simulink model "acc_test"  (R2020a)
settings: Solver=VariableStepAuto  StartTime=0.0  StopTime=6594  RelTol=1e-3
values from neighbouring files (symbols this model uses):
  max_CE_power = 100    [Parallel_script.m]    (also in Series_script.m = 60)
  max_EG_power = 40    [Series_script.m]
  max_EM_power = 84    [Parallel_script.m]    (also in Series_script.m = 90)
  max_SOC = 0.60    (= 0.6)    [Parallel_script.m]    (also in Series_script.m = 0.5)
  min_SOC = 0.35    [Parallel_script.m]    (also in Series_script.m = 0.3)
  Series_add_Mass = 150    [Series_script.m]
  T_CE_max = p_me_max*V_d/(2*pi*2)    [Parallel_script.m]    (also in Series_script.m)
  T_EG_max = T_EG_max * max_EG_power*1000/max_EG_power_old    [Series_script.m]
  T_EM_max = T_EM_max * max_EM_power*1000/max_EM_power_old    [Parallel_script.m]    (also in Series_script.m)
  V_Mass = 1920    [Parallel_script.m]    (also in Series_script.m)
undefined symbols (not defined in the file or in its folder): eta_EG_map, eta_EM_map, H_u, P_aux, P_CE_cutoff, P_CE_idle, T_CE_cutoff, theta_CE, theta_EM, V_CE_map, w_CE_idle, w_CE_max, w_CE_upper, w_EG_row, w_EG_upper, w_EM_row, w_EM_upper
libraries: qss_tb_library x7
settings Model: Creator=Rahul Pai  LastModifiedBy=Rahul Pai

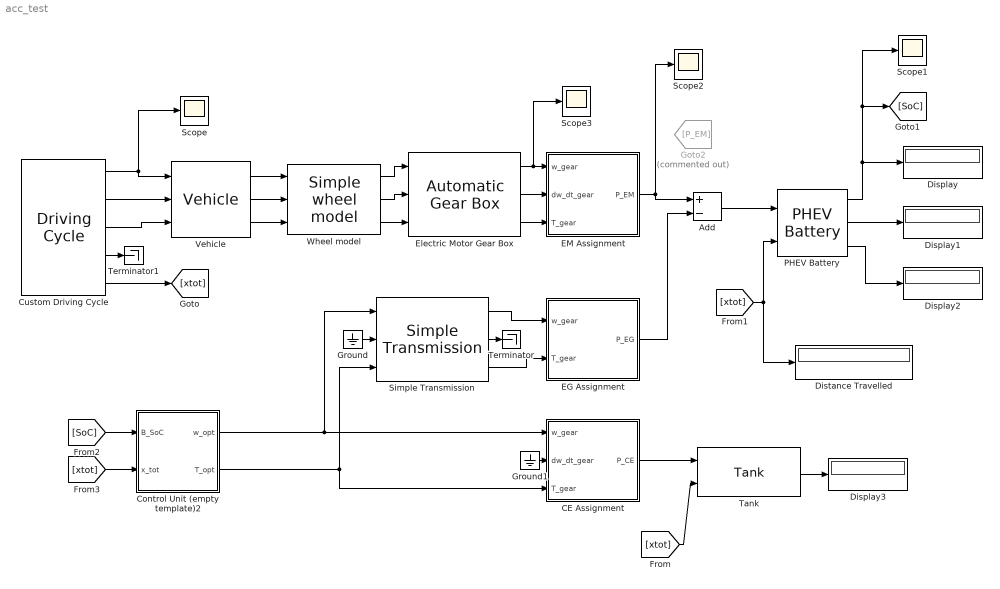
== system acc_test ==
  Add : Sum  Inputs=+-
  CE Assignment : Subsystem  Tag=combustion engine  AncestorBlock=qss_tb_library/Energy Converter/CE Assignment  mask(Combustion Engine (based on consumption map)){engine_type=Gasoline, P_ice=max_CE_power, ENABLE_FUEL_CUTOFF=on}
      mask prompts: engine_type "Engine type"; P_ice "Power [kW]"; ENABLE_FUEL_CUTOFF "Enable fuel cutoff"
      mask help:
      | This block simulates the behaviour of a combustion engine. The block is based on consumption maps for medium sized passenger cars.
      |
      | NA Gasoline:
      | max power @ 5000 rpm
      | max torque @ 3000 rpm
      |
      | Small Diesel:
      | max power @ 4500 rpm
      | max torque @ 2000 rpm
      |
      | Large Diesel:
      | max power @ 1500 rpm
      | max torque @ 1500 rpm
      |
      |
      | Input:
      | =====
      | 	w_gear	Speed of the fly wheel [rad/s]
      | 	dw_dt_gear	Acceleration of the fly wheel [rad/s^2]
      | 	T_gear	Torque on the fly wheel [Nm]
      |
      | Output:
      | ======
      | 	P_CE	Fuel power consumed by the combustion engine [W]
      mask init:
      | init_AssCE_map;
      mask TypeOptions engine_type: Gasoline | Small Diesel | Large Diesel
  Control Unit (empty template)2 : Subsystem  Tag=control unit  AncestorBlock=|  mask(Control Unit){}
      | qss_tb_library/Controller/Control Unit
      | (empty template)
      mask help:
      | This block gives the user the opportunity to design his/her own control unit.
      |
      | The user can define the inputs and outputs  by himself/herself.
  Custom Driving Cycle : qss_tb_library/Driving Cycle/Driving Cycle  Tag=cycle  cyclename1=assignment2_custom_cycle_full  stepsize=1  autostop=on
  Display{,1..3} (4 alike) : Display
  Distance Travelled : Display
      settings: Format=decimal (Stored Integer)
  EG Assignment : Subsystem  AncestorBlock=qss_tb_library/Energy Converter/EG Assignment  mask(Electric Generator){P_eg=max_EG_power}
      mask prompts: P_eg "Maximum mechanical power [kW]"
      mask help:
      | This block simulates the behaviour of an electric generator. The block is based on an efficiency map.
      |
      | Input:
      | =====
      | 	w_gear	Speed of the generator [rad/s]
      | 	T_gear	Torque of the generator [Nm]
      |
      | Output:
      | ======
      | 	P_EG	Electric power of the generator [W]
      |
      | Generator map:
      | ======
      | The generator map file must contain the following variables:
      | eta_EG_map		% Efficiency map                    [-]
      | w_EG_row                        % Generator speed range             [rad/s]
      | T_EG_col		% Generator torque range            [Nm]
      | w_EG_max		% Maximum generator speed           [rad/s]
      | T_EG_max		% Maximum generator torque          [Nm]
      |
      | ======
      mask init:
      | init_EG_ass;
  EM Assignment : Subsystem  AncestorBlock=qss_tb_library/Energy Converter/EM Assignment  mask(Electric Motor){P_em=max_EM_power}
      mask prompts: P_em "Power [kW]"
      mask help:
      | This block simulates the behaviour of an electric motor. The block is based on an efficiency map. The map is located in the Data/EnergyConvertter/ElectricMotor directory.
      |
      | Maximum speed och the electric motor is 6000 rpm
      | Field weakening region starts at 1500 rpm
      | Maximum mechanical power is at 2150 rpm
      | The maximum torque is 5.98 Nm/kW multiplied with the power you select.
      |
      | Input:
      | =====
      | 	w_gear	Speed of the motor [rad/s]
      | 	dw_dt_gear	Acceleration of the motor [rad/s^2]
      | 	T_gear	Torque of the motor [Nm]
      |
      | Output:
      | ======
      | 	P_EM	Electric Power consumed by the  motor [W]
      mask init:
      | init_EM_ass;
  Electric Motor Gear Box : qss_tb_library/Gear System/Automatic Gear Box  Tag=transmission  nog=Gears  i=gear_ratio  i_diff=diff_gear  gearon=gear_up  gearoff=gear_down  d=V_wheel_dia  e_GT=gear_eff  P_GT0=gear_idling_loss  w_wheel_min=1
  Goto2 : Goto  Commented=on  GotoTag=P_EM
  Ground : Ground
  Ground1 : Ground
  PHEV Battery : qss_tb_library/Energy Buffer/PHEV Battery  Tag=battery  cell_series=N_series  cell_parallel=N_parallel  Q_BT_IC_rel=Init_SoC
  Scope{,1..3} (4 alike) : Scope
  Simple Transmission : qss_tb_library/Gear System/Simple Transmission  Tag=simple transmission  gear_ratio=EM_gear_ratio  e_GT=EM_gear_eta  P_GT0=EM_idling_loss  w_wheel_min=1
  Tank : qss_tb_library/Energy Source/Tank  Tag=tank  fuel=Gasoline  flag_cold_start=on
  Terminator : Terminator
  Terminator1 : Terminator
  Vehicle : qss_tb_library/Vehicle/Vehicle  Tag=vehicle  m_f=V_Mass+Series_add_Mass  A_f=V_area  cw=V_d  mu=V_RRC  k_inertia=V_Rotating
  Wheel model : qss_tb_library/Vehicle/Simple wheel model  Tag=simple transmission  d_wheel=V_wheel_dia
  wires:
  Custom Driving Cycle/4 -> Terminator1/1
  EG Assignment/1(P_EG) -> Add/2
  EM Assignment/1(P_EM) -> Add/1, Scope2/1
  Control Unit (empty template)2/2(T_opt) -> Simple Transmission/3, CE Assignment/3(T_gear)
  Simple Transmission/2 -> Terminator/1
  [xtot] -> Control Unit (empty template)2/2(x_tot)
  Wheel model/3 -> Electric Motor Gear Box/3
  Add/1 -> PHEV Battery/1
  Simple Transmission/3 -> EG Assignment/2(T_gear)
  Control Unit (empty template)2/1(w_opt) -> Simple Transmission/1, CE Assignment/1(w_gear)
  [SoC] -> Control Unit (empty template)2/1(B_SoC)
  [xtot] -> PHEV Battery/2, Distance Travelled/1
  Ground1/1 -> CE Assignment/2(dw_dt_gear)
  PHEV Battery/3 -> Display2/1
  Custom Driving Cycle/5 -> [xtot]
  Custom Driving Cycle/3 -> Vehicle/3
  Vehicle/3 -> Wheel model/3
  Electric Motor Gear Box/2 -> EM Assignment/2(dw_dt_gear)
  Simple Transmission/1 -> EG Assignment/1(w_gear)
  CE Assignment/1(P_CE) -> Tank/1
  Wheel model/2 -> Electric Motor Gear Box/2
  Tank/1 -> Display3/1
  Electric Motor Gear Box/3 -> EM Assignment/3(T_gear)
  Vehicle/2 -> Wheel model/2
  Wheel model/1 -> Electric Motor Gear Box/1
  [xtot] -> Tank/2
  Electric Motor Gear Box/1 -> Scope3/1, EM Assignment/1(w_gear)
  PHEV Battery/1 -> Scope1/1, [SoC], Display/1
  PHEV Battery/2 -> Display1/1
  Custom Driving Cycle/2 -> Vehicle/2
  Custom Driving Cycle/1 -> Scope/1, Vehicle/1
  Vehicle/1 -> Wheel model/1
  Ground/1 -> Simple Transmission/2

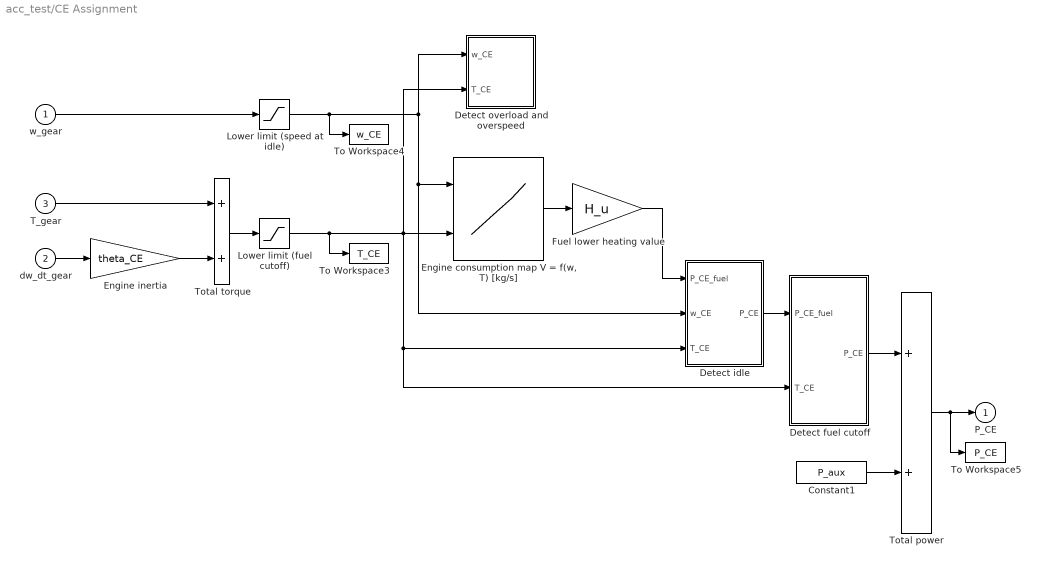
== system acc_test/CE Assignment ==
  w_gear : Inport
  dw_dt_gear : Inport  Port=2
  T_gear : Inport  Port=3
  Constant1 : Constant  Value=P_aux
  Detect fuel cutoff : Subsystem
  Detect idle : Subsystem
  Detect overload and overspeed : Subsystem
  "Engine consumption map V = f(w, T) [kg/s]" : Lookup2D  RowIndex=w_CE_row  ColumnIndex=T_CE_col  Table=V_CE_map
  Engine inertia : Gain  Gain=theta_CE  SaturateOnIntegerOverflow=on  OutDataTypeStr=Inherit: Same as input  ParamDataTypeStr=Inherit: Same as input
  Fuel lower heating value : Gain  Gain=H_u  SaturateOnIntegerOverflow=on  OutDataTypeStr=Inherit: Same as input  ParamDataTypeStr=Inherit: Same as input
  Lower limit (fuel cutoff) : Saturate  UpperLimit=inf  LowerLimit=T_CE_cutoff
  Lower limit (speed at idle) : Saturate  UpperLimit=inf  LowerLimit=w_CE_idle
  To Workspace3 : ToWorkspace  VariableName=T_CE  SampleTime=-1
  To Workspace4 : ToWorkspace  VariableName=w_CE  SampleTime=-1
  To Workspace5 : ToWorkspace  VariableName=P_CE  SampleTime=-1
  Total power : Sum  InputSameDT=on  SaturateOnIntegerOverflow=on  OutDataTypeStr=Inherit: Same as first input
  Total torque : Sum  InputSameDT=on  SaturateOnIntegerOverflow=on  OutDataTypeStr=Inherit: Same as first input
  P_CE : Outport  InitialOutput=0
  wires:
  T_gear/1 -> Total torque/1
  dw_dt_gear/1 -> Engine inertia/1
  Total torque/1 -> Lower limit (fuel cutoff)/1
  Engine inertia/1 -> Total torque/2
  Lower limit (speed at idle)/1 -> Detect overload and overspeed/1(w_CE), Detect idle/2(w_CE), "Engine consumption map V = f(w, T) [kg/s]"/1, To Workspace4/1
  w_gear/1 -> Lower limit (speed at idle)/1
  Fuel lower heating value/1 -> Detect idle/1(P_CE_fuel)
  Detect idle/1(P_CE) -> Detect fuel cutoff/1(P_CE_fuel)
  "Engine consumption map V = f(w, T) [kg/s]"/1 -> Fuel lower heating value/1
  Detect fuel cutoff/1(P_CE) -> Total power/1
  Total power/1 -> P_CE/1, To Workspace5/1
  Constant1/1 -> Total power/2
  Lower limit (fuel cutoff)/1 -> Detect overload and overspeed/2(T_CE), "Engine consumption map V = f(w, T) [kg/s]"/2, Detect idle/3(T_CE), Detect fuel cutoff/2(T_CE), To Workspace3/1

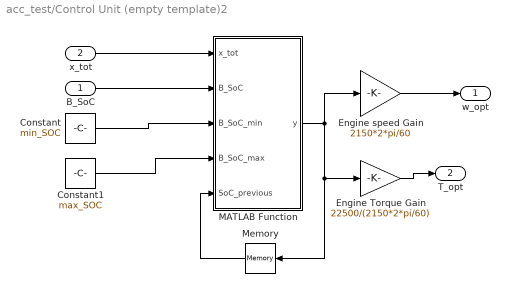
== system acc_test/Control Unit (empty template)2 ==
  B_SoC : Inport
  x_tot : Inport  Port=2
  Constant : Constant  Value=min_SOC
  Constant1 : Constant  Value=max_SOC
  Engine Torque Gain : Gain  Gain=22500/(2150*2*pi/60)
  Engine speed Gain : Gain  Gain=2150*2*pi/60
  MATLAB Function : MATLAB Function  TreatAsAtomicUnit=on
  Memory : Memory
  w_opt : Outport  InitialOutput=0
  T_opt : Outport  Port=2  InitialOutput=0
  wires:
  Memory/1 -> MATLAB Function/5(SoC_previous)
  x_tot/1 -> MATLAB Function/1(x_tot)
  Engine Torque Gain/1 -> T_opt/1
  Constant/1 -> MATLAB Function/3(B_SoC_min)
  Engine speed Gain/1 -> w_opt/1
  B_SoC/1 -> MATLAB Function/2(B_SoC)
  MATLAB Function/1(y) -> Engine Torque Gain/1, Memory/1, Engine speed Gain/1
  Constant1/1 -> MATLAB Function/4(B_SoC_max)

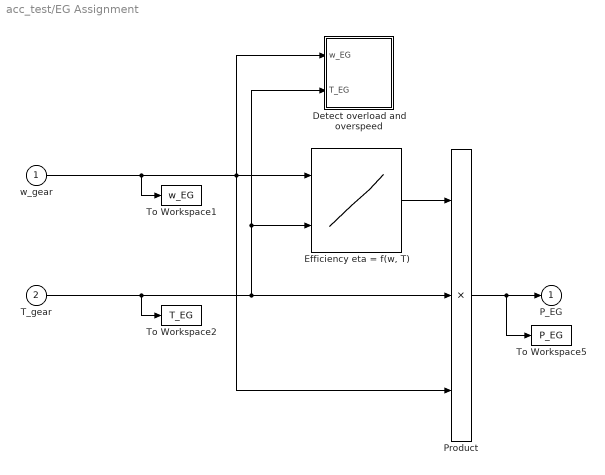
== system acc_test/EG Assignment ==
  w_gear : Inport
  T_gear : Inport  Port=2
  Detect overload and overspeed : Subsystem
  "Efficiency eta = f(w, T)" : Lookup2D  RowIndex=w_EG_row  ColumnIndex=T_EG_col  Table=eta_EG_map
  Product : Product  Inputs=3  InputSameDT=on  RndMeth=Zero  SaturateOnIntegerOverflow=on  OutDataTypeStr=Inherit: Same as first input
  To Workspace1 : ToWorkspace  VariableName=w_EG  SampleTime=-1
  To Workspace2 : ToWorkspace  VariableName=T_EG  SampleTime=-1
  To Workspace5 : ToWorkspace  VariableName=P_EG  SampleTime=-1
  P_EG : Outport  InitialOutput=0
  wires:
  w_gear/1 -> To Workspace1/1, Detect overload and overspeed/1(w_EG), "Efficiency eta = f(w, T)"/1, Product/3
  Product/1 -> To Workspace5/1, P_EG/1
  "Efficiency eta = f(w, T)"/1 -> Product/1
  T_gear/1 -> To Workspace2/1, Detect overload and overspeed/2(T_EG), "Efficiency eta = f(w, T)"/2, Product/2

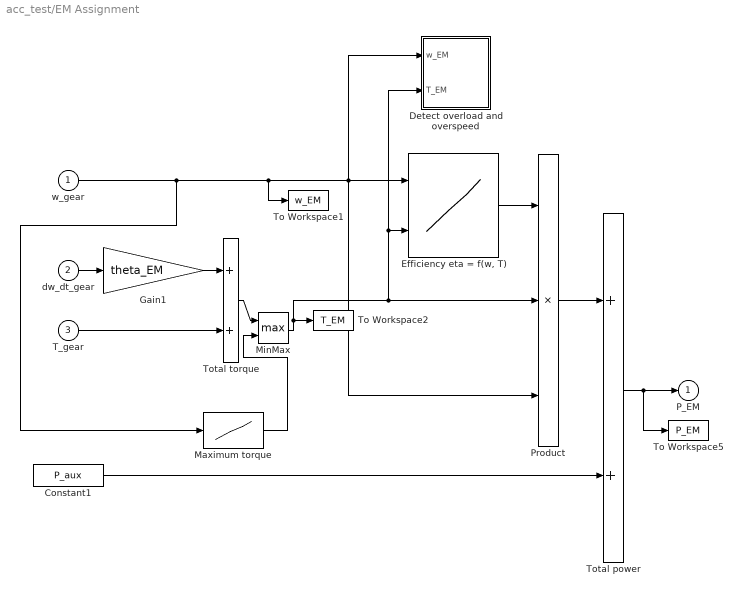
== system acc_test/EM Assignment ==
  w_gear : Inport
  dw_dt_gear : Inport  Port=2
  T_gear : Inport  Port=3
  Constant1 : Constant  Value=P_aux
  Detect overload and overspeed : Subsystem
  "Efficiency eta = f(w, T)" : Lookup2D  RowIndex=w_EM_row  ColumnIndex=T_EM_col  Table=eta_EM_map
  Gain1 : Gain  Gain=theta_EM  SaturateOnIntegerOverflow=on  OutDataTypeStr=Inherit: Same as input  ParamDataTypeStr=Inherit: Same as input
  Maximum torque : Lookup  InputValues=w_EM_row  Table=-T_EM_max  SaturateOnIntegerOverflow=on
  MinMax : MinMax  Function=max  Inputs=2
  Product : Product  Inputs=3  InputSameDT=on  RndMeth=Zero  SaturateOnIntegerOverflow=on  OutDataTypeStr=Inherit: Same as first input
  To Workspace1 : ToWorkspace  VariableName=w_EM  SampleTime=-1
  To Workspace2 : ToWorkspace  VariableName=T_EM  SampleTime=-1
  To Workspace5 : ToWorkspace  VariableName=P_EM  SampleTime=-1
  Total power : Sum  InputSameDT=on  SaturateOnIntegerOverflow=on  OutDataTypeStr=Inherit: Same as first input
  Total torque : Sum  InputSameDT=on  SaturateOnIntegerOverflow=on  OutDataTypeStr=Inherit: Same as first input
  P_EM : Outport  InitialOutput=0
  wires:
  Total power/1 -> To Workspace5/1, P_EM/1
  Product/1 -> Total power/1
  Constant1/1 -> Total power/2
  MinMax/1 -> Product/2, "Efficiency eta = f(w, T)"/2, Detect overload and overspeed/2(T_EM), To Workspace2/1
  Gain1/1 -> Total torque/1
  T_gear/1 -> Total torque/2
  dw_dt_gear/1 -> Gain1/1
  "Efficiency eta = f(w, T)"/1 -> Product/1
  w_gear/1 -> Maximum torque/1, To Workspace1/1, Product/3, "Efficiency eta = f(w, T)"/1, Detect overload and overspeed/1(w_EM)
  Total torque/1 -> MinMax/1
  Maximum torque/1 -> MinMax/2

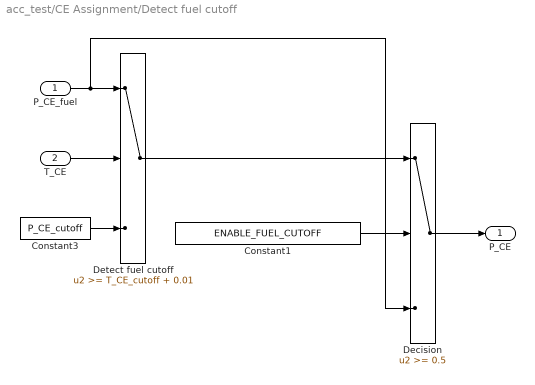
== system acc_test/CE Assignment/Detect fuel cutoff ==
  P_CE_fuel : Inport
  T_CE : Inport  Port=2
  Constant1 : Constant  Value=ENABLE_FUEL_CUTOFF
  Constant3 : Constant  Value=P_CE_cutoff
  Decision : Switch  Threshold=0.5
  Detect fuel cutoff : Switch  Threshold=T_CE_cutoff + 0.01  SaturateOnIntegerOverflow=on  InputSameDT=on
  P_CE : Outport
  wires:
  Constant3/1 -> Detect fuel cutoff/3
  T_CE/1 -> Detect fuel cutoff/2
  P_CE_fuel/1 -> Detect fuel cutoff/1, Decision/3
  Detect fuel cutoff/1 -> Decision/1
  Constant1/1 -> Decision/2
  Decision/1 -> P_CE/1

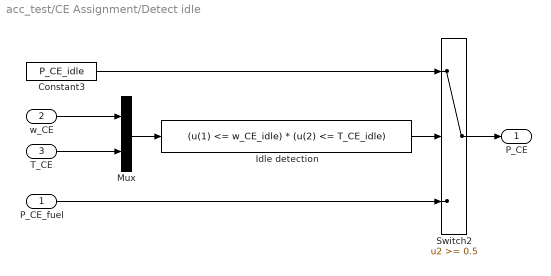
== system acc_test/CE Assignment/Detect idle ==
  P_CE_fuel : Inport
  w_CE : Inport  Port=2
  T_CE : Inport  Port=3
  Constant3 : Constant  Value=P_CE_idle
  Idle detection : Fcn  Expr=(u(1) <= w_CE_idle) * (u(2) <= T_CE_idle)
  Mux : Mux  Inputs=2
  Switch2 : Switch  Threshold=0.5  SaturateOnIntegerOverflow=on  InputSameDT=on
  P_CE : Outport  InitialOutput=0
  wires:
  Mux/1 -> Idle detection/1
  T_CE/1 -> Mux/2
  w_CE/1 -> Mux/1
  Idle detection/1 -> Switch2/2
  P_CE_fuel/1 -> Switch2/3
  Switch2/1 -> P_CE/1
  Constant3/1 -> Switch2/1

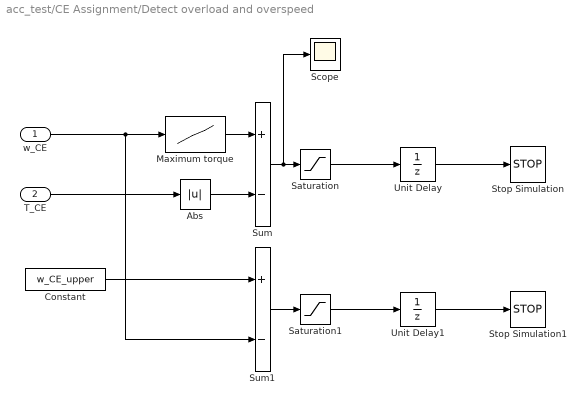
== system acc_test/CE Assignment/Detect overload and overspeed ==
  w_CE : Inport
  T_CE : Inport  Port=2
  Abs : Abs  SaturateOnIntegerOverflow=on
  Constant : Constant  Value=w_CE_upper
  Maximum torque : Lookup  InputValues=w_CE_max  Table=T_CE_max  SaturateOnIntegerOverflow=on
  Saturation : Saturate  UpperLimit=0  LowerLimit=-inf
  Saturation1 : Saturate  UpperLimit=0  LowerLimit=-inf
  Scope : Scope
  Stop Simulation : Stop
  Stop Simulation1 : Stop
  Sum : Sum  Inputs=+-  InputSameDT=on  SaturateOnIntegerOverflow=on  OutDataTypeStr=Inherit: Same as first input
  Sum1 : Sum  Inputs=+-  InputSameDT=on  SaturateOnIntegerOverflow=on  OutDataTypeStr=Inherit: Same as first input
  Unit Delay : UnitDelay  SampleTime=-1  HasFrameUpgradeWarning=on
  Unit Delay1 : UnitDelay  SampleTime=-1  HasFrameUpgradeWarning=on
  wires:
  Sum/1 -> Scope/1, Saturation/1
  w_CE/1 -> Maximum torque/1, Sum1/2
  T_CE/1 -> Abs/1
  Maximum torque/1 -> Sum/1
  Abs/1 -> Sum/2
  Saturation/1 -> Unit Delay/1
  Constant/1 -> Sum1/1
  Sum1/1 -> Saturation1/1
  Saturation1/1 -> Unit Delay1/1
  Unit Delay/1 -> Stop Simulation/1
  Unit Delay1/1 -> Stop Simulation1/1

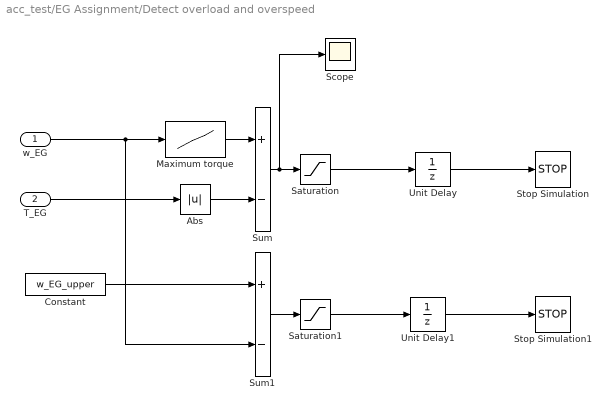
== system acc_test/EG Assignment/Detect overload and overspeed ==
  w_EG : Inport
  T_EG : Inport  Port=2
  Abs : Abs  SaturateOnIntegerOverflow=on
  Constant : Constant  Value=w_EG_upper
  Maximum torque : Lookup  InputValues=w_EG_row  Table=T_EG_max  SaturateOnIntegerOverflow=on
  Saturation : Saturate  UpperLimit=0  LowerLimit=-inf
  Saturation1 : Saturate  UpperLimit=0  LowerLimit=-inf
  Scope : Scope
  Stop Simulation : Stop
  Stop Simulation1 : Stop
  Sum : Sum  Inputs=+-  InputSameDT=on  SaturateOnIntegerOverflow=on  OutDataTypeStr=Inherit: Same as first input
  Sum1 : Sum  Inputs=+-  InputSameDT=on  SaturateOnIntegerOverflow=on  OutDataTypeStr=Inherit: Same as first input
  Unit Delay : UnitDelay  SampleTime=-1  HasFrameUpgradeWarning=on
  Unit Delay1 : UnitDelay  SampleTime=-1  HasFrameUpgradeWarning=on
  wires:
  Saturation1/1 -> Unit Delay1/1
  Sum1/1 -> Saturation1/1
  Constant/1 -> Sum1/1
  Saturation/1 -> Unit Delay/1
  Abs/1 -> Sum/2
  Maximum torque/1 -> Sum/1
  T_EG/1 -> Abs/1
  w_EG/1 -> Sum1/2, Maximum torque/1
  Sum/1 -> Scope/1, Saturation/1
  Unit Delay/1 -> Stop Simulation/1
  Unit Delay1/1 -> Stop Simulation1/1

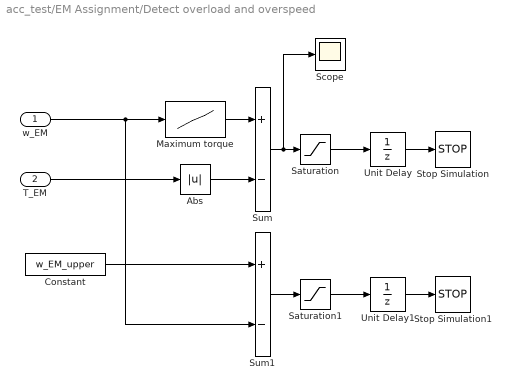
== system acc_test/EM Assignment/Detect overload and overspeed ==
  w_EM : Inport
  T_EM : Inport  Port=2
  Abs : Abs  SaturateOnIntegerOverflow=on
  Constant : Constant  Value=w_EM_upper
  Maximum torque : Lookup  InputValues=w_EM_row  Table=T_EM_max  SaturateOnIntegerOverflow=on
  Saturation : Saturate  UpperLimit=0  LowerLimit=-inf
  Saturation1 : Saturate  UpperLimit=0  LowerLimit=-inf
  Scope : Scope
  Stop Simulation : Stop
  Stop Simulation1 : Stop
  Sum : Sum  Inputs=+-  InputSameDT=on  SaturateOnIntegerOverflow=on  OutDataTypeStr=Inherit: Same as first input
  Sum1 : Sum  Inputs=+-  InputSameDT=on  SaturateOnIntegerOverflow=on  OutDataTypeStr=Inherit: Same as first input
  Unit Delay : UnitDelay  SampleTime=-1  HasFrameUpgradeWarning=on
  Unit Delay1 : UnitDelay  SampleTime=-1  HasFrameUpgradeWarning=on
  wires:
  Sum/1 -> Scope/1, Saturation/1
  w_EM/1 -> Maximum torque/1, Sum1/2
  T_EM/1 -> Abs/1
  Maximum torque/1 -> Sum/1
  Abs/1 -> Sum/2
  Saturation/1 -> Unit Delay/1
  Constant/1 -> Sum1/1
  Sum1/1 -> Saturation1/1
  Saturation1/1 -> Unit Delay1/1
  Unit Delay/1 -> Stop Simulation/1
  Unit Delay1/1 -> Stop Simulation1/1

== matlab function acc_test/Control Unit (empty template)2/MATLAB Function ==
  data: x_tot input; y output; B_SoC input; B_SoC_min input; B_SoC_max input; SoC_previous input
function y = fcn(x_tot,B_SoC,B_SoC_min,B_SoC_max,SoC_previous)
if x_tot==1
    SoC=0;
else
    if B_SoC>B_SoC_max
        SoC=0;
    else
        if B_SoC<=B_SoC_min
            SoC=1;
        else
            SoC=SoC_previous;
        end
    end
end
y = SoC;
